simulink model "PlanarDynamics"  (R2018b)
settings: Solver=FixedStepAuto  StartTime=0.0  StopTime=50  FixedStep=0.025  RelTol=1e-3
InitFcn:
  | loadThrusterData
undefined symbols (not defined in the file or in its folder): DiscIntNeverNeededParam
settings Model: Creator=Andy  LastModifiedBy=barthal
settings DataIOCC: SaveOutput=off  SaveTime=off
settings ModelReferenceCC: ModelReferenceNumInstancesAllowed=Single
settings RTWCC: GenCodeOnly=on

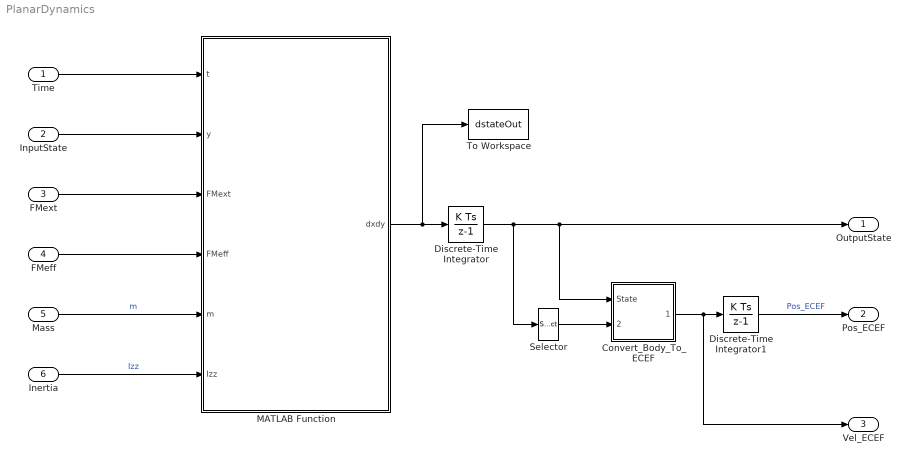
== system PlanarDynamics ==
  Time : Inport  OutDataTypeStr=double  PortDimensions=1  SampleTime=[0.025000000000000001,0]
  InputState : Inport  Port=2  OutDataTypeStr=double  PortDimensions=9  SampleTime=[0.025000000000000001,0]
  FMext : Inport  Port=3  OutDataTypeStr=double  PortDimensions=3
  FMeff : Inport  Port=4  OutDataTypeStr=double  PortDimensions=3  SampleTime=[0.025000000000000001,0]
  Mass : Inport  Port=5  OutDataTypeStr=double  PortDimensions=1  SampleTime=[0.025000000000000001,0]
  Inertia : Inport  Port=6  OutDataTypeStr=double  PortDimensions=1  SampleTime=[0.025000000000000001,0]
  Convert_Body_To_ECEF : Subsystem
  Discrete-Time Integrator : DiscreteIntegrator  SampleTime=-1  ICPrevOutput=DiscIntNeverNeededParam  ICPrevScaledInput=DiscIntNeverNeededParam
  Discrete-Time Integrator1 : DiscreteIntegrator  SampleTime=-1  ICPrevOutput=DiscIntNeverNeededParam  ICPrevScaledInput=DiscIntNeverNeededParam
  MATLAB Function : MATLAB Function  TreatAsAtomicUnit=on
  Selector : Selector  InputPortWidth=9  IndexOptions=Index vector (dialog)  Indices=[4:6]  OutputSizes=1
  To Workspace : ToWorkspace  VariableName=dstateOut  SaveFormat=Timeseries  SampleTime=-1
  OutputState : Outport  OutDataTypeStr=double  PortDimensions=9  SampleTime=[0.025000000000000001,0]
  Pos_ECEF : Outport  Port=2  OutDataTypeStr=double  PortDimensions=3  SampleTime=[0.025000000000000001,0]
  Vel_ECEF : Outport  Port=3  OutDataTypeStr=double  PortDimensions=3  SampleTime=[0.025000000000000001,0]
  wires:
  MATLAB Function/1(dxdy) -> To Workspace/1, Discrete-Time Integrator/1
  FMext/1 -> MATLAB Function/3(FMext)
  Selector/1 -> Convert_Body_To_ECEF/2(Vec_Body)
  FMeff/1 -> MATLAB Function/4(FMeff)
  Discrete-Time Integrator/1 -> Convert_Body_To_ECEF/1(State), OutputState/1, Selector/1
  Time/1 -> MATLAB Function/1(t)
  Mass/1 -> MATLAB Function/5(m)  "m"
  InputState/1 -> MATLAB Function/2(y)
  Convert_Body_To_ECEF/1(Vec_ECEF) -> Discrete-Time Integrator1/1, Vel_ECEF/1
  Discrete-Time Integrator1/1 -> Pos_ECEF/1  "Pos_ECEF"
  Inertia/1 -> MATLAB Function/6(Izz)  "Izz"

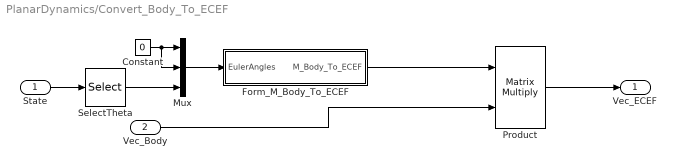
== system PlanarDynamics/Convert_Body_To_ECEF ==
  State : Inport  PortDimensions=9
  Vec_Body : Inport  Port=2  PortDimensions=3
  Constant : Constant  Value=0
  Form_M_Body_To_ECEF : Subsystem
  Mux : Mux  Inputs=3
  Product : Product  Multiplication=Matrix(*)
  SelectTheta : Selector  InputPortWidth=9  IndexOptions=Index vector (dialog)  Indices=3  OutputSizes=1
  Vec_ECEF : Outport  PortDimensions=3
  wires:
  Product/1 -> Vec_ECEF/1
  Vec_Body/1 -> Product/2
  Form_M_Body_To_ECEF/1(M_Body_To_ECEF) -> Product/1
  State/1 -> SelectTheta/1
  Mux/1 -> Form_M_Body_To_ECEF/1(EulerAngles)
  Constant/1 -> Mux/2, Mux/1
  SelectTheta/1 -> Mux/3

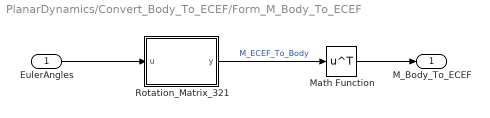
== system PlanarDynamics/Convert_Body_To_ECEF/Form_M_Body_To_ECEF ==
  EulerAngles : Inport
  Math Function : Math  Operator=transpose  SaturateOnIntegerOverflow=on
  Rotation_Matrix_321 : MATLAB Function  TreatAsAtomicUnit=on
  M_Body_To_ECEF : Outport
  wires:
  Rotation_Matrix_321/1(y) -> Math Function/1  "M_ECEF_To_Body"
  Math Function/1 -> M_Body_To_ECEF/1
  EulerAngles/1 -> Rotation_Matrix_321/1(u)

== matlab function PlanarDynamics/Convert_Body_To_ECEF/Form_M_Body_To_ECEF/Rotation_Matrix_321 ==
  data: u input; y output
function y = fcn(u)
% Form a 3-2-1 Euler angle rotation matrix
% 
% Inputs: u        rotation angles in 1,2,3 order 3x1
%
% Output: y        rotation matrix 3x3
%
% Assumptions and Limitations:
%    Angles are input in radians
%
% References:
%    Wie, Bong. Space vehicle dynamics and control. 
%    American Institute of Aeronautics and Astronautics, 2008.
%
% Author: Andrew Barth
%
% Modification History:
%    May 14 2019 - Initial version
%

% Form aliases
c1 = cos(u(1));
s1 = sin(u(1));
c2 = cos(u(2));
s2 = sin(u(2));
c3 = cos(u(3));
s3 = sin(u(3));

% Form the rotation matrix
y = [ c2*c3           c2*s3          -s2; ...
      s1*s2*c3-c1*s3  s1*s2*s3+c1*c3  s1*c2; ...
      c1*s2*c3+s1*s3  c1*s2*s3-s1*c3  c1*c2];

== matlab function PlanarDynamics/MATLAB Function ==
  data: t input; dxdy output; y input; FMext input; FMeff input; m input; Izz input
function dxdy = callplanarEOM(t,y,FMext,FMeff,m,Izz)

 dxdy = planarEOM(t,y,FMext,FMeff,m,Izz);
